simulink subsystem "Vehicle1D_Custom_refsub"  (R2026a)
settings: Solver=VariableStepAuto
PreLoadFcn:
  | defineBus_Rotational
libraries: nesl_utility x6, fl_lib x1
settings Model: Creator=isaacito  LastModifiedBy=isaacito
settings SimscapeCC: SimscapeNominalValues="[{\"value\":\"1\",\"unit\":\"A\"},{\"value\":\"1\",\"unit\":\"bar\"},{\"value\":\"1\",\"unit\":\"cm^2\"},{\"value\":\"1\",\"unit\":\"cm^3/s\"},{\"value\":\"1\",\"unit\":\"kJ/kg\"},{\"value\":\"1\",\"unit\":\"kW\"},{\"value\":\"1\",\"unit\":\"l\"},{\"value\":\"1\",\"unit\":\"N\"},{\"value\":\"1\",\"unit\":\"N*m\"},{\"value\":\"1\",\"unit\":\"V\"}]"  SimscapeLogType=none  SimscapeLogDataHistory=5000.0

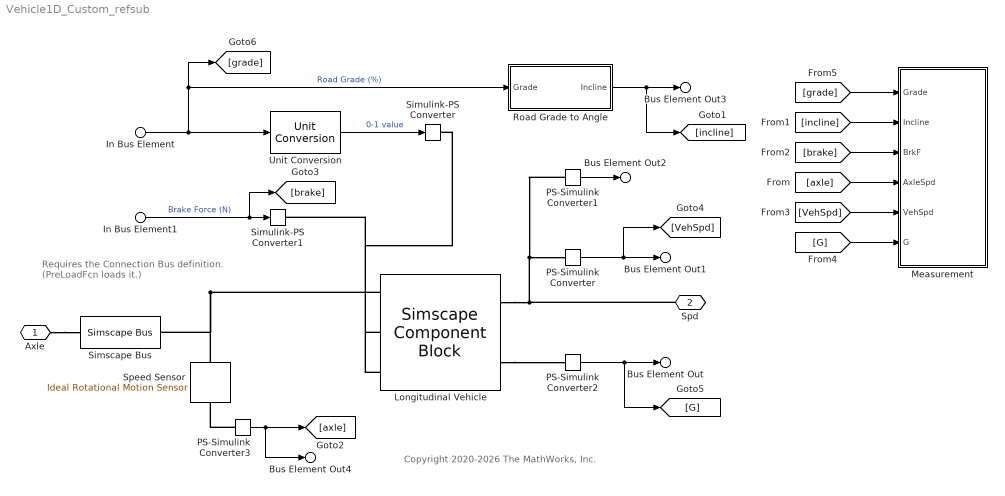
== system Vehicle1D_Custom_refsub ==
  note: Requires the Connection Bus definition.
      | (PreLoadFcn loads it.)
  note: Copyright 2020-2026 The MathWorks, Inc.
  In Bus Element : Inport  PortName=Inputs  Element=RoadGrade
      settings: AttributesFormatString=%<Unit>
  In Bus Element1 : Inport  PortName=Inputs  Element=BrakeForce
      settings: AttributesFormatString=%<Unit>
  Longitudinal Vehicle : SimscapeComponentBlock  SourceFile=Vehicle1D_Custom  ComponentPath=Vehicle1D_Custom  ComponentVariants="[\"Vehicle1D_Custom\"]"  ComponentVariantNames="[\"Vehicle1D_Custom\"]"  ClassName=Vehicle1D_Custom  SchemaVersion=1  grav=9.81 m/s^2  M_e=vehicle.mass_kg kg  R_tire=vehicle.tireRollingRadius_m m  A_rl=vehicle.roadLoadA_N N  B_rl=0 N*hr/km  C_rl=vehicle.roadLoadC_N_per_kph2 N*hr^2/km^2  V_1=smoothing.vehicle_speedThreshold_kph km/hr  w_1=smoothing.vehicle_axleSpeedThreshold_rpm rpm  V_x_specify=on  V_x_priority=High  V_x=initial.vehicle_speed_kph km/hr  V_x_nominal_specify=off  V_x_nominal_value=1  V_x_nominal_unit=km/hr
      settings: AttributesFormatString=%<V_x>  CopyFcn=simscape.sscblock.internal.componentBlockCallback(gcbh,'COPY')  PreCopyFcn=simscape.sscblock.internal.componentBlockCallback(gcbh,'PRECOPY')  PreDeleteFcn=simscape.sscblock.internal.componentBlockCallback(gcbh,'PREDELETE')  LogSimulationData=on
      mask Type: Custom Longitudinal Vehicle
  Measurement : Subsystem
  PS-Simulink Converter : nesl_utility/PS-Simulink Converter  PhysicalDomain=network_engine_domain  SubClassName=ps_output  LeftPortType=input  RightPortType=output  PseudoPeriodic=off  Frequencies=[]  VectorFormat=1-D array  Unit=km/hr  AffineConversion=off
  PS-Simulink Converter1 : nesl_utility/PS-Simulink Converter  PhysicalDomain=network_engine_domain  SubClassName=ps_output  LeftPortType=input  RightPortType=output  PseudoPeriodic=off  Frequencies=[]  VectorFormat=1-D array  Unit=mph  AffineConversion=off
  PS-Simulink Converter2 : nesl_utility/PS-Simulink Converter  PhysicalDomain=network_engine_domain  SubClassName=ps_output  LeftPortType=input  RightPortType=output  PseudoPeriodic=off  Frequencies=[]  VectorFormat=1-D array  Unit=1  AffineConversion=off
  PS-Simulink Converter3 : nesl_utility/PS-Simulink Converter  PhysicalDomain=network_engine_domain  SubClassName=ps_output  LeftPortType=input  RightPortType=output  PseudoPeriodic=off  Frequencies=[]  VectorFormat=1-D array  Unit=rpm  AffineConversion=off
  Road Grade to Angle : Subsystem
  Simscape Bus : SimscapeBus  HierarchyStrings=AngSpd  ConnectionType=Bus: Bus_Rotational
      settings: AttributesFormatString=%<ConnectionType>
  Simulink-PS Converter : nesl_utility/Simulink-PS Converter  PhysicalDomain=network_engine_domain  SubClassName=ps_input  LeftPortType=input  RightPortType=output  PseudoPeriodic=off  Frequencies=[]  NoiseDistribution=none  NoiseParameters=[]  Unit=1  AffineConversion=off  FilteringAndDerivatives=filter  SimscapeFilterOrder=1  InputFilterTimeConstant=0.001  UdotUserProvided=0
  Simulink-PS Converter1 : nesl_utility/Simulink-PS Converter  PhysicalDomain=network_engine_domain  SubClassName=ps_input  LeftPortType=input  RightPortType=output  PseudoPeriodic=off  Frequencies=[]  NoiseDistribution=none  NoiseParameters=[]  Unit=N  AffineConversion=off  FilteringAndDerivatives=filter  SimscapeFilterOrder=1  InputFilterTimeConstant=0.001  UdotUserProvided=0
  Speed Sensor : fl_lib/Mechanical/Mechanical Sensors/Ideal Rotational Motion Sensor  reference=foundation.enum.MeasurementReference.absolute  acceleration_port=false  velocity_port=true  position_port=false  wrap_angle=simscape.enum.onoff.off  offset=0 rad
  Unit Conversion : UnitConversion  OutputType=Inherit: Inherit via back propagation
  Axle : PMIOPort  Side=Left
  Spd : PMIOPort  Port=2  Side=Right
  Bus Element Out : Outport  PortName=Info  Element=G
      settings: AttributesFormatString=%<Unit>
  Bus Element Out1 : Outport  PortName=Info  Element=VehSpdKph
      settings: AttributesFormatString=%<Unit>
  Bus Element Out2 : Outport  PortName=Info  Element=VehSpdMph
      settings: AttributesFormatString=%<Unit>
  Bus Element Out3 : Outport  PortName=Info  Element=Incline
      settings: AttributesFormatString=%<Unit>
  Bus Element Out4 : Outport  PortName=Info  Element=AxleSpd
      settings: AttributesFormatString=%<Unit>
  wires:
  PS-Simulink Converter/1 -> [VehSpd], Bus Element Out1/1
  PS-Simulink Converter2/1 -> [G], Bus Element Out/1
  In Bus Element/1 -> Unit Conversion/1, [grade], Road Grade to Angle/1(Grade)  "Road Grade (%)"
  In Bus Element1/1 -> [brake], Simulink-PS Converter1/1  "Brake Force (N)"
  Unit Conversion/1 -> Simulink-PS Converter/1  "0-1 value"
  PS-Simulink Converter1/1 -> Bus Element Out2/1
  Road Grade to Angle/1(Incline) -> Bus Element Out3/1, [incline]
  [incline] -> Measurement/2(Incline)
  [brake] -> Measurement/3(BrkF)
  [axle] -> Measurement/4(AxleSpd)
  [VehSpd] -> Measurement/5(VehSpd)
  [G] -> Measurement/6(G)
  [grade] -> Measurement/1(Grade)
  PS-Simulink Converter3/1 -> Bus Element Out4/1, [axle]
  connections:
  Longitudinal Vehicle/RConn1 -- Spd/RConn1 -- PS-Simulink Converter1/LConn1 -- PS-Simulink Converter/LConn1
  Longitudinal Vehicle/LConn1 -- Speed Sensor/LConn1 -- Simscape Bus/LConn1
  Longitudinal Vehicle/RConn2 -- PS-Simulink Converter2/LConn1
  Longitudinal Vehicle/LConn3 -- Simulink-PS Converter/RConn1
  Longitudinal Vehicle/LConn2 -- Simulink-PS Converter1/RConn1
  Axle/RConn1 -- Simscape Bus/RConn1
  PS-Simulink Converter3/LConn1 -- Speed Sensor/RConn1

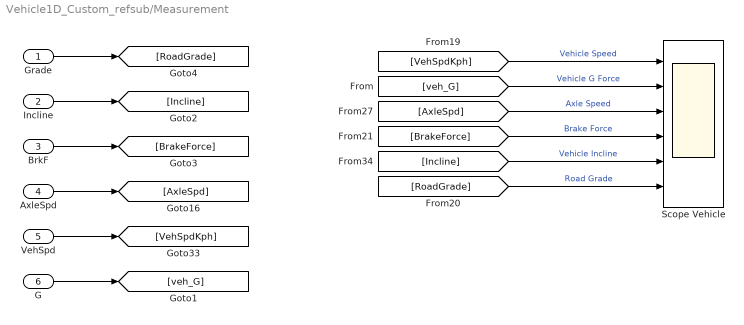
== system Vehicle1D_Custom_refsub/Measurement ==
  Grade : Inport
  Incline : Inport  Port=2
  BrkF : Inport  Port=3
  AxleSpd : Inport  Port=4
  VehSpd : Inport  Port=5
  G : Inport  Port=6
  Scope Vehicle : Scope  NumInputPorts=6
      settings: ActiveDisplayYMinimum=-12.00926  ActiveDisplayYMaximum=102.7511
  wires:
  [VehSpdKph] -> Scope Vehicle/1  "Vehicle Speed"
  [veh_G] -> Scope Vehicle/2  "Vehicle G Force"
  AxleSpd/1 -> [AxleSpd]
  VehSpd/1 -> [VehSpdKph]
  G/1 -> [veh_G]
  Incline/1 -> [Incline]
  BrkF/1 -> [BrakeForce]
  [AxleSpd] -> Scope Vehicle/3  "Axle Speed"
  [BrakeForce] -> Scope Vehicle/4  "Brake Force"
  [Incline] -> Scope Vehicle/5  "Vehicle Incline"
  [RoadGrade] -> Scope Vehicle/6  "Road Grade"
  Grade/1 -> [RoadGrade]

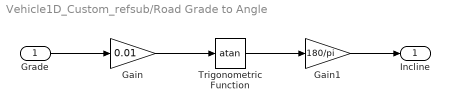
== system Vehicle1D_Custom_refsub/Road Grade to Angle ==
  Grade : Inport  Unit=%
      settings: AttributesFormatString=%<Unit>
  Gain : Gain  Gain=0.01
  Gain1 : Gain  Gain=180/pi
  Trigonometric Function : Trigonometry  Operator=atan
  Incline : Outport  Unit=deg
      settings: AttributesFormatString=%<Unit>
  wires:
  Gain1/1 -> Incline/1
  Trigonometric Function/1 -> Gain1/1
  Grade/1 -> Gain/1
  Gain/1 -> Trigonometric Function/1
